simulink model "linear_feedback_without_dist_2019"  (R2019a)
settings: Solver=VariableStepAuto  StartTime=0.0  StopTime=6  RelTol=1e-3
undefined symbols (not defined in the file): A_l, B_l, C_l, initial_condition, K_slow
settings Model: Creator=mahdi  LastModifiedBy=mahdi
settings DebuggingCC: SFMachineParentedDataDiag=error

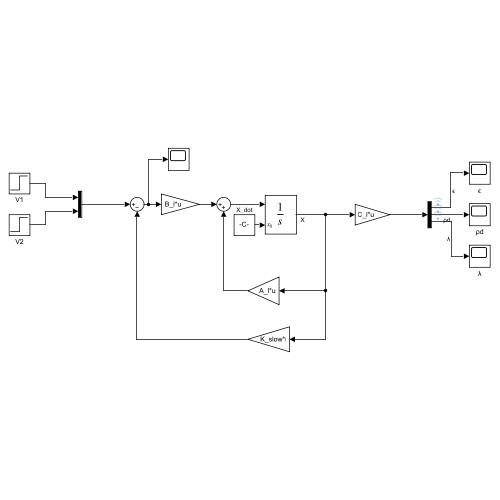
[thumbnail: Simulink's stored preview of the top-level diagram]
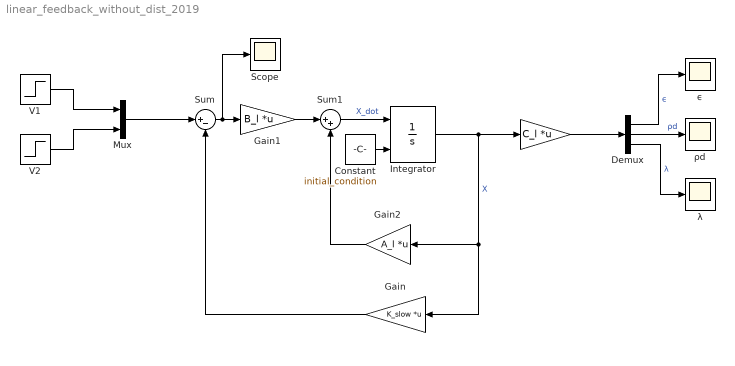
== system linear_feedback_without_dist_2019 ==
  " " : Gain  Gain=C_l  Multiplication=Matrix(K*u)
  Constant : Constant  Value=initial_condition
  Demux : Demux  Outputs=3
  Gain : Gain  Gain=K_slow  Multiplication=Matrix(K*u)
  Gain1 : Gain  Gain=B_l  Multiplication=Matrix(K*u)
  Gain2 : Gain  Gain=A_l  Multiplication=Matrix(K*u)
  Integrator : Integrator  InitialConditionSource=external  InitialCondition=initial_condition
  Mux : Mux  Inputs=2
  Scope : Scope
  Sum : Sum  Inputs=|+-
  Sum1 : Sum  Inputs=|++
  V1 : Step  Time=0  After=0  SampleTime=0
  V2 : Step  After=0  SampleTime=0
  λ : Scope
  ρd : Scope
  ϵ : Scope
  wires:
  Sum/1 -> Scope/1, Gain1/1
  Gain/1 -> Sum/2
  Gain1/1 -> Sum1/1
  Sum1/1 -> Integrator/1  "X_dot"
  Integrator/1 -> " "/1, Gain/1, Gain2/1  "X"
  " "/1 -> Demux/1
  Gain2/1 -> Sum1/2
  V2/1 -> Mux/2
  V1/1 -> Mux/1
  Mux/1 -> Sum/1
  Demux/1 -> ϵ/1  "ϵ"
  Demux/2 -> ρd/1  "ρd"
  Demux/3 -> λ/1  "λ"
  Constant/1 -> Integrator/2
